simulink model "BlockDiagram"  (R2017a)
settings: Solver=VariableStepAuto  StartTime=0.0  StopTime=10.0  RelTol=1e-3
values from neighbouring files (symbols this model uses):
  dm = 3.8e-6    (= 3.8e-06)    [ex2.m]
  J = (n*n*Jr + Jl) / n    (= 3.7300072)    [ex2.m]
  Ke = Kt / 9.55    (= 0.00729842931937)    [ex2.m]
  Kt = 69.7e-3    (= 0.0697)    [ex2.m]
  n = 5    [ex2.m]
  R = 112    [ex2.m]
settings Model: Creator=99641  LastModifiedBy=99641

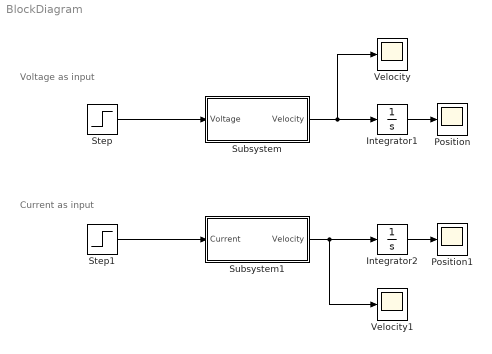
== system BlockDiagram ==
  note: Current as input
  note: Voltage as input
  Integrator1 : Integrator
  Integrator2 : Integrator
  Position : Scope
  Position1 : Scope
  Step : Step  SampleTime=0
  Step1 : Step  SampleTime=0
  Subsystem : Subsystem
  Subsystem1 : Subsystem
  Velocity : Scope
  Velocity1 : Scope
  wires:
  Step/1 -> Subsystem/1(Voltage)
  Subsystem/1("Velocity ") -> Velocity/1, Integrator1/1
  Integrator1/1 -> Position/1
  Step1/1 -> Subsystem1/1(Current)
  Integrator2/1 -> Position1/1
  Subsystem1/1("Velocity ") -> Integrator2/1, Velocity1/1

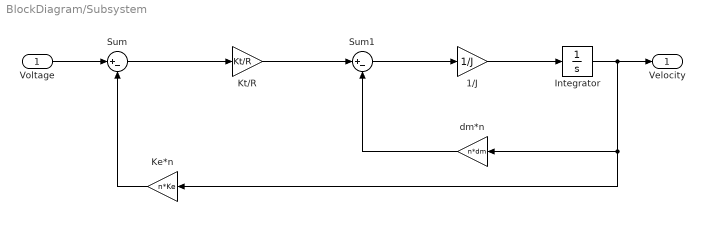
== system BlockDiagram/Subsystem ==
  Voltage : Inport
  1/J : Gain  Gain=1/J
  Integrator : Integrator
  Ke*n : Gain  Gain=n*Ke
  Kt/R : Gain  Gain=Kt/R
  Sum : Sum  Inputs=|+-
  Sum1 : Sum  Inputs=|+-
  dm*n : Gain  Gain=n*dm
  "Velocity " : Outport
  wires:
  Voltage/1 -> Sum/1
  Sum/1 -> Kt/R/1
  Sum1/1 -> 1/J/1
  Kt/R/1 -> Sum1/1
  1/J/1 -> Integrator/1
  Integrator/1 -> Ke*n/1, dm*n/1, "Velocity "/1
  dm*n/1 -> Sum1/2
  Ke*n/1 -> Sum/2

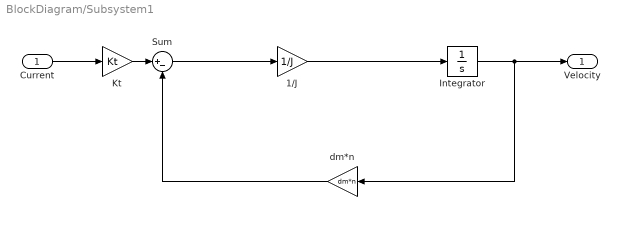
== system BlockDiagram/Subsystem1 ==
  Current : Inport
  1/J : Gain  Gain=1/J
  Integrator : Integrator
  Kt : Gain  Gain=Kt
  Sum : Sum  Inputs=|+-
  dm*n : Gain  Gain=dm*n
  "Velocity " : Outport
  wires:
  dm*n/1 -> Sum/2
  Integrator/1 -> "Velocity "/1, dm*n/1
  1/J/1 -> Integrator/1
  Sum/1 -> 1/J/1
  Current/1 -> Kt/1
  Kt/1 -> Sum/1
